simulink model "model"  (R2024b)
settings: Solver=VariableStepAuto  StartTime=0.0  StopTime=5  RelTol=1e-3
values from neighbouring files (symbols this model uses):
  elevationTolerance = 15e-2    (= 0.15)    [ortho_setup.m]
  nthFrame = 100    [ortho_setup.m]
  pitchTolerance = 2    [ortho_setup.m]
  rollVelocityTolerance = 1e-4    (= 0.0001)    [ortho_setup.m]
  targetUAVElevation = 80    [ortho_setup.m]
undefined symbols (not defined in the file or in its folder): Sim3dSensor
libraries: visionsinks x3, uavalgslib x2, sim3dcameralib x2, uavsim3dlib x2, sim3dlib x1
settings Model: Creator=jacob  LastModifiedBy=Jacob

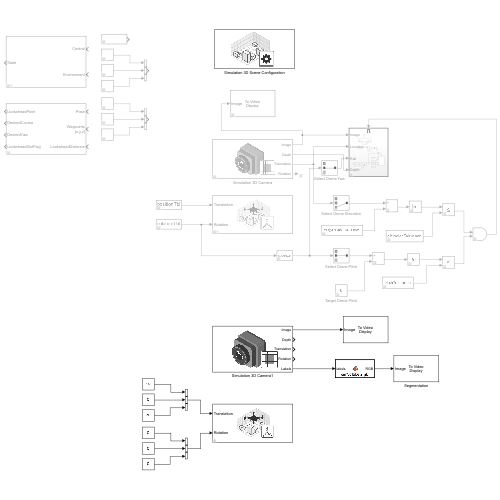
[thumbnail: Simulink's stored preview of the top-level diagram]
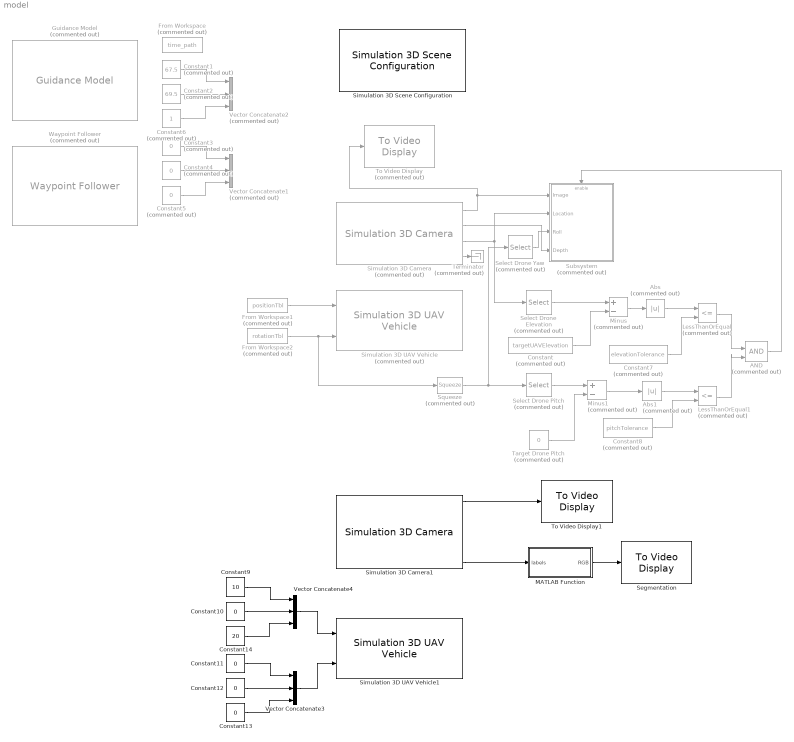
== system model ==
  AND : Logic  Commented=on  IconShape=distinctive  AllPortsSameDT=off  OutDataTypeStr=boolean
  Abs : Abs  Commented=on  SaturateOnIntegerOverflow=off
  Abs1 : Abs  Commented=on  SaturateOnIntegerOverflow=off
  Constant : Constant  Commented=on  Value=targetUAVElevation
  Constant1 : Constant  Commented=on  Value=67.5
  Constant{10..13} (4 alike) : Constant  Value=0
  Constant14 : Constant  Value=20
  Constant2 : Constant  Commented=on  Value=69.5
  Constant3 : Constant  Commented=on  Value=0
  Constant4 : Constant  Commented=on  Value=0
  Constant5 : Constant  Commented=on  Value=0
  Constant6 : Constant  Commented=on
  Constant7 : Constant  Commented=on  Value=elevationTolerance
  Constant8 : Constant  Commented=on  Value=pitchTolerance
  Constant9 : Constant  Value=10
  From Workspace : FromWorkspace  Commented=on  VariableName=time_path
  From Workspace1 : FromWorkspace  Commented=on  VariableName=positionTbl
  From Workspace2 : FromWorkspace  Commented=on  VariableName=rotationTbl
  Guidance Model : uavalgslib/Guidance Model  Commented=on  ModelType=MultirotorGuidance  SpecifiedDataType=double  SimulateUsing=Interpreted execution  InitialWorldPositionMultirotor=[0; 0; 0]  InitialWorldVelocityMultirotor=[0; 0; 0]  InitialEulerZYXMultirotor=[0; 0; 0]  InitialBodyAngularRateRPYMultirotor=[0; 0; 0]  InitialThrustMultirotor=0  InitialNorthFixedWing=0  InitialEastFixedWing=0  InitialHeightFixedWing=0  InitialAirSpeedFixedWing=0  InitialHeadingAngleFixedWing=0  InitialFlightPathAngleFixedWing=0  InitialRollAngleFixedWing=0  InitialRollAngleRateFixedWing=0  PDRollMultirotor=[3402.97,116.67]  PDPitchMultirotor=[3402.97, 116.67]  PYawRateMultirotor=1950  PThrustMultirotor=3900  MassMultirotor=0.1  PHeightFixedWing=3.9  PHeadingAngleFixedWing=3.9  PFlightPathAngleFixedWing=39  PDRollFixedWing=[3402.97, 116.67]  PAirSpeedFixedWing=1  FlightPathAngleLimitsFixedWing=[-pi/2, pi/2]  StateBusName='MultirotorGuidanceStateBus'  ControlBusName='MultirotorGuidanceControlBus'  EnvironmentBusName='MultirotorGuidanceEnvironmentBus'  DataType=double
  LessThanOrEqual : RelationalOperator  Commented=on  Operator=<=  OutDataTypeStr=boolean  RndMeth=Simplest  InputSameDT=off
  LessThanOrEqual1 : RelationalOperator  Commented=on  Operator=<=  OutDataTypeStr=boolean  RndMeth=Simplest  InputSameDT=off
  MATLAB Function : MATLAB Function  TreatAsAtomicUnit=on
  Minus : Sum  Commented=on  Inputs=+-
  Minus1 : Sum  Commented=on  Inputs=+-
  Segmentation : visionsinks/To Video Display  windowSizeMode=Normal  openAtMdlStart=on  fullScreen=off  videoWindowX=536805376  videoWindowY=536805376  saveWindowSize=off  videoWindowWidth=1024  videoWindowHeight=1024  inputColorFormat=RGB  inputType=Obsolete  imagePorts=One multidimensional signal  OutputDevice=On-screen video monitor  dataOrg=Column-major  isWindowOpen=off
  Select Drone Elevation : Selector  Commented=on  InputPortWidth=3  IndexOptions=Index vector (dialog)  Indices=[3]  OutputSizes=1
  Select Drone Pitch : Selector  Commented=on  InputPortWidth=3  IndexOptions=Index vector (dialog)  Indices=[2]  OutputSizes=1
  Select Drone Yaw : Selector  Commented=on  InputPortWidth=3  IndexOptions=Index vector (dialog)  Indices=[2]  OutputSizes=1
  Simulation 3D Camera : sim3dcameralib/Simulation 3D Camera  Priority=1  Commented=on  sensorTag=Sim3dSensor�  sensorId=1  sensorName=Sim3dSensor�  vehTagList={'Quadrotor';'Scene Origin'}  vehTag=Quadrotor  mountLoc=Origin  offsetFlag=on  tmountOffset=[0, 0, 0.1]  extTmount=off  rmountOffset=[0, 90, 0]  extRmount=off  FocalLength=[1109, 1109]  OpticalCenter=[640, 360]  ImageSize=[1024, 1024]  RadialDistortion=[0, 0]  TangentialDistortion=[0, 0]  SensorSkew=0  DepthOutportEnabled=on  SemanticOutportEnabled=off  TransformOutportEnabled=on  SampleTime=-1  mountPoint=[0 0 0.1]  mountOrientation=[0 -90 0]  aMode=4  ID=1
      settings: LibrarySourceBlock=uavsim3dlib/Simulation 3D Camera
  Simulation 3D Camera1 : sim3dcameralib/Simulation 3D Camera  Priority=1  sensorTag=Sim3dSensor�  sensorId=2  sensorName=Sim3dSensor�  vehTagList={'Quadrotor';'Scene Origin';'SimulinkVehicle1'}  vehTag=Quadrotor  mountLoc=Origin  offsetFlag=on  tmountOffset=[0, 0, 0.1]  extTmount=off  rmountOffset=[0, 90, 0]  extRmount=off  FocalLength=[1109, 1109]  OpticalCenter=[640, 360]  ImageSize=[1024, 1024]  RadialDistortion=[0, 0]  TangentialDistortion=[0, 0]  SensorSkew=0  DepthOutportEnabled=on  SemanticOutportEnabled=on  TransformOutportEnabled=on  SampleTime=-1  mountPoint=[0 0 0.1]  mountOrientation=[0 -90 0]  aMode=4  ID=2
      settings: LibrarySourceBlock=uavsim3dlib/Simulation 3D Camera
  Simulation 3D Scene Configuration : sim3dlib/Simulation 3D Scene Configuration  Priority=0  ProjectFormat=Unreal Editor  SceneDesc=US city block  ProjectName=C:\Program Files\MATLAB\R2024b\toolbox\shared\sim3d_projects\automotive_project_windows\UE\WindowsNoEditor\VehicleSimulation.exe  ScenePath=/Game/Maps/USCityBlock  UEProjPath=C:\project\AutoVrtlEnv\AutoVrtlEnv.uproject  EnableOpenDRIVE=off  vehTagList={'Custom';'Quadrotor';'Scene Origin'}  vehTag=Quadrotor  FreeCameraInitialTranslation=[67.5, -60, 2]  FreeCameraDefaultInitialTranslation=[-6, 0, 2]  FreeCameraInitialRotation=[0, 0, 0]  FreeCameraDefaultInitialRotation=[0, -15, 0]  OpVisEn=off  Ts=1/60  EnableWindow=on  EnableRemoteAccess=off  EnableWeather=off  SunAzimuth=90  SunAltitude=40.0  EnableGeospatialSun=off  Latitude=0  Longitude=0  Date=2023-01-01  Time=10:30:00  GeoTimeZone=-5.0  SunDaylightSaving=off  wind=1  clouds=10  EnableVolumetricClouds=off  CloudCoverage=0  CloudAltitude=6  fog=0  rain=0  RaindropsEffect=off  SnowDensity=0  EnableGeospatial=off  UseTrueOrigin=off  OriginHeight=200  OriginLatitude=40.744652  OriginLongitude=-73.988864  MapStyle=Aerial  AdditionalAssetIDs=[]  UseAdvancedSunSky=off  SolarTime=11  TimeZone=-5  Day=21  Month=9  Year=2022  UseDaylightSavingTime=on  DSTStartDay=10  DSTStartMonth=3  DSTEndDay=3  DSTEndMonth=11  DSTSwitchHour=2  sensorTag=MainCamera1  sensorId=1  sensorName=MainCamera1  mountLoc=Origin  offsetFlag=off  tmountOffset=[0, 0, 0]  rmountOffset=[0, 0, 0]  HorizontalResolution=1280  VerticalResolution=720  HorizontalFOV=60  mountPoint=[0 0 0]  mountOrientation=[0 0 0]  aMode=4  ID=1  GeoTrigger=Inactive
      settings: LibrarySourceBlock=uavsim3dlib/Simulation 3D Scene Configuration
  Simulation 3D UAV Vehicle : uavsim3dlib/Simulation 3D UAV Vehicle  Priority=-1  Commented=on  Mesh=Quadrotor  MeshPath=/MathWorksUAVContent/UAVs/HexaRotorUAV/HexaRotor.HexaRotor  Color=Black  ActorName=Quadrotor1  UseGlobalFrame=off  InitialTranslation=[67.5 -69.5 0]  InitialRotation=[0 0 0]  InitialTranslationGlobal=[0 0 0]  InitialGeoOrigin=[0 0 0]  InitialRotationGlobal=[0 0 0]  SampleTime=-1  ActorType=SimulinkVehicle  ID=C  aMode=4  ActorTag=Quadrotor1
  Simulation 3D UAV Vehicle1 : uavsim3dlib/Simulation 3D UAV Vehicle  Priority=-1  Mesh=Quadrotor  MeshPath=/MathWorksUAVContent/UAVs/HexaRotorUAV/HexaRotor.HexaRotor  Color=Black  ActorName=Quadrotor  UseGlobalFrame=off  InitialTranslation=[0 0 0]  InitialRotation=[0 0 0]  InitialTranslationGlobal=[0 0 0]  InitialGeoOrigin=[0 0 0]  InitialRotationGlobal=[0 0 0]  SampleTime=-1  ActorType=SimulinkVehicle  ID=C  aMode=4  ActorTag=Quadrotor
  Squeeze : Squeeze  Commented=on
  Subsystem : Subsystem  Commented=on
  Target Drone Pitch : Constant  Commented=on  Value=0
  Terminator : Terminator  Commented=on
  To Video Display : visionsinks/To Video Display  Commented=on  windowSizeMode=Normal  openAtMdlStart=on  fullScreen=off  videoWindowX=536805376  videoWindowY=536805376  saveWindowSize=off  videoWindowWidth=1280  videoWindowHeight=720  inputColorFormat=RGB  inputType=Obsolete  imagePorts=One multidimensional signal  OutputDevice=On-screen video monitor  dataOrg=Column-major  isWindowOpen=off
  To Video Display1 : visionsinks/To Video Display  windowSizeMode=Normal  openAtMdlStart=on  fullScreen=off  videoWindowX=536805376  videoWindowY=536805376  saveWindowSize=off  videoWindowWidth=1280  videoWindowHeight=720  inputColorFormat=RGB  inputType=Obsolete  imagePorts=One multidimensional signal  OutputDevice=On-screen video monitor  dataOrg=Column-major  isWindowOpen=off
  Vector Concatenate1 : Concatenate  Commented=on  NumInputs=3
  Vector Concatenate2 : Concatenate  Commented=on  NumInputs=3
  Vector Concatenate3 : Concatenate  NumInputs=3
  Vector Concatenate4 : Concatenate  NumInputs=3
  Waypoint Follower : uavalgslib/Waypoint Follower  Commented=on  UAVType=multirotor  StartFrom=first  TransitionRadiusSource=internal  TransitionRadius=10  MinLookaheadDistance=0.1  HoverAtLastWaypoint=off  YawInput=off  ShowCrossTrackErrorOutput=off  ShowStatusOutput=off  SimulateUsing=Interpreted execution
  wires:
  Simulation 3D Camera/1 -> To Video Display/1, Subsystem/1(Image)
  Constant4/1 -> Vector Concatenate1/2
  Constant3/1 -> Vector Concatenate1/1
  Constant5/1 -> Vector Concatenate1/3
  Constant1/1 -> Vector Concatenate2/1
  Constant6/1 -> Vector Concatenate2/3
  Constant2/1 -> Vector Concatenate2/2
  From Workspace1/1 -> Simulation 3D UAV Vehicle/1
  From Workspace2/1 -> Squeeze/1, Simulation 3D UAV Vehicle/2
  Simulation 3D Camera/3 -> Subsystem/2(Location), Select Drone Elevation/1
  Select Drone Elevation/1 -> Minus/1
  Constant/1 -> Minus/2
  Minus/1 -> Abs/1
  Constant7/1 -> LessThanOrEqual/2
  Abs/1 -> LessThanOrEqual/1
  Squeeze/1 -> Select Drone Yaw/1, Select Drone Pitch/1
  Select Drone Pitch/1 -> Minus1/1
  Target Drone Pitch/1 -> Minus1/2
  Minus1/1 -> Abs1/1
  Abs1/1 -> LessThanOrEqual1/1
  Constant8/1 -> LessThanOrEqual1/2
  LessThanOrEqual/1 -> AND/1
  LessThanOrEqual1/1 -> AND/2
  AND/1 -> Subsystem/Enable
  Simulation 3D Camera/4 -> Terminator/1
  Select Drone Yaw/1 -> Subsystem/3(Roll)
  Simulation 3D Camera/2 -> Subsystem/4(Depth)
  Constant13/1 -> Vector Concatenate3/3
  Constant9/1 -> Vector Concatenate4/1
  Constant14/1 -> Vector Concatenate4/3
  Constant10/1 -> Vector Concatenate4/2
  Constant12/1 -> Vector Concatenate3/2
  Constant11/1 -> Vector Concatenate3/1
  Vector Concatenate4/1 -> Simulation 3D UAV Vehicle1/1
  Vector Concatenate3/1 -> Simulation 3D UAV Vehicle1/2
  Simulation 3D Camera1/1 -> To Video Display1/1
  Simulation 3D Camera1/5 -> MATLAB Function/1(labels)
  MATLAB Function/1(RGB) -> Segmentation/1

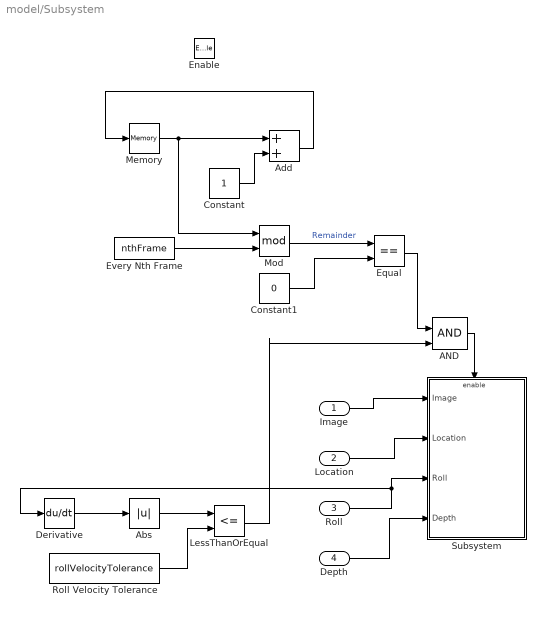
== system model/Subsystem ==
  Image : Inport
  Location : Inport  Port=2
  Roll : Inport  Port=3
  Depth : Inport  Port=4
  Enable : EnablePort
  AND : Logic  IconShape=distinctive  AllPortsSameDT=off  OutDataTypeStr=boolean
  Abs : Abs  SaturateOnIntegerOverflow=off
  Add : Sum
  Constant : Constant
  Constant1 : Constant  Value=0
  Derivative : Derivative
  Equal : RelationalOperator  Operator===  OutDataTypeStr=boolean  RndMeth=Simplest  InputSameDT=off
  Every Nth Frame : Constant  Value=nthFrame
  LessThanOrEqual : RelationalOperator  Operator=<=  OutDataTypeStr=boolean  RndMeth=Simplest  InputSameDT=off
  Memory : Memory
  Mod : Math  Operator=mod
  Roll Velocity Tolerance : Constant  Value=rollVelocityTolerance
  Subsystem : Subsystem
  wires:
  Memory/1 -> Add/1, Mod/1
  Constant/1 -> Add/2
  Add/1 -> Memory/1
  Every Nth Frame/1 -> Mod/2
  Constant1/1 -> Equal/2
  Mod/1 -> Equal/1  "Remainder"
  Derivative/1 -> Abs/1
  Abs/1 -> LessThanOrEqual/1
  Roll Velocity Tolerance/1 -> LessThanOrEqual/2
  LessThanOrEqual/1 -> AND/2
  Equal/1 -> AND/1
  Image/1 -> Subsystem/1(Image)
  Location/1 -> Subsystem/2(Location)
  Roll/1 -> Derivative/1, Subsystem/3(Roll)
  AND/1 -> Subsystem/Enable
  Depth/1 -> Subsystem/4(Depth)

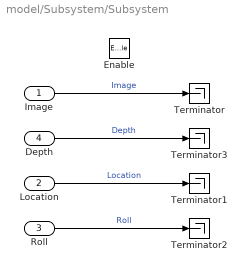
== system model/Subsystem/Subsystem ==
  Image : Inport
  Location : Inport  Port=2
  Roll : Inport  Port=3
  Depth : Inport  Port=4
  Enable : EnablePort
  Terminator{,1..3} (4 alike) : Terminator
  wires:
  Image/1 -> Terminator/1  "Image"
  Location/1 -> Terminator1/1  "Location"
  Roll/1 -> Terminator2/1  "Roll"
  Depth/1 -> Terminator3/1  "Depth"

== matlab function model/MATLAB Function ==
  data: labels input; RGB output
function RGB = sim3dlabel2rgb(labels)
% Convert semantic segmentation map captured during 3D simulation to RGB
% color image.

% Declare label2rgb function.
coder.extrinsic('label2rgb');

% Preallocate memory for RGB matrix.
RGB = coder.nullcopy(zeros(size(labels,1),size(labels,2),3,class(labels)));

% Define colormap using 3D simulation label IDs.
cmap = sim3dColormap;

% Convert labels to RGB color image.
RGB = label2rgb(labels, cmap);
